simulink model "printer"  (R2017b)
settings: Solver=ode45  StartTime=0.0  StopTime=3  FixedStep=1e-4  MaxStep=1e-4  RelTol=1e-3  EnableMultiTasking=on
PreLoadFcn:
  | CONSTANTS
  | DEFAULT
  | System
  | Control
InitFcn:
  | CONSTANTS
  | DEFAULT
  | System
  | Control
values from neighbouring files (symbols this model uses):
  BackEMF0 = Q0(13)    [System.m]
  BackEMF1 = Q1(13)    [System.m]
  DegPerRad = 180/pi    (= 57.2957795131)    [CONSTANTS.m]    (also in kinematics_circle_MEGA.m = 57.3; kinematics_circle_fast_MEGA.m = 57.3; kinematics_circle_slow_MEGA.m = 57.3; kinematics_triangle_MEGA.m = 57.3)
  Elec0d = [Q0(11) Q0(10)]    [System.m]
  Elec0n = [1]    [System.m]
  Elec1d = [Q1(11) Q1(10)]    [System.m]
  Elec1n = [1]    [System.m]
  Height = 0.1    [CONSTANTS.m]
  Mech0d = [J0 B0]    [System.m]
  Mech0n = [1]    [System.m]
  Mech1d = [J1 B1]    [System.m]
  Mech1n = [1]    [System.m]
  NomI0 = Q0(6)    [System.m]
  NomI1 = Q1(6)    [System.m]
  PID0 = [0.178 8.83 0.0785]    [Control.m]
  PID1 = [Kp1 Ki1 Kd1]    [Control.m]
  StallI0 = Q0(8)    [System.m]
  StallI1 = Q1(8)    [System.m]
  StFric0 = 0.0024    [System.m]
  TConst0 = Q0(12)    [System.m]
  TConst1 = Q1(12)    [System.m]
undefined symbols (not defined in the file or in its folder): Amp1d, Amp1n, AmpSat1, JntSat1, Sens0, Sens1, SensSat0, SensSat1
libraries: simulink x14
settings Model: Creator=Leos  LastModifiedBy=cgx19
settings DataIOCC: SaveFormat=Array
settings OptimizationCC: ExpressionDepthLimit=2147483647  LifeSpan=inf
settings DebuggingCC: UnderspecifiedInitializationDetection=Classic  MergeDetectMultiDrivingBlocksExec=none  SolverPrmCheckMsg=warning  FcnCallInpInsideContextMsg=warning  StateNameClashWarn=warning  SFUnexpectedBacktrackingDiag=warning  SFNoUnconditionalDefaultTransitionDiag=warning  SFExecutionAtInitializationDiag=none
settings HardwareCC: ProdBitPerPointer=32  ProdBitPerSizeT=32  ProdBitPerPtrDiffT=32  ProdLargestAtomicFloat=None  ProdIntDivRoundTo=Undefined  ProdEndianess=Unspecified  ProdWordSize=32  ProdHWDeviceType=32-bit Generic
settings ModelReferenceCC: PropagateSignalLabelsOutOfModel=off
settings CodeAppCC: StateflowObjectComments=on
settings GRTTargetCC: TargetLangStandard=C89/C90 (ANSI)  GeneratePreprocessorConditionals=Disable all  CombineOutputUpdateFcns=off  GRTInterface=on
settings ConfigComp: CovMetricSettings=dw  CovHtmlReporting=on  CovSaveCumulativeToWorkspaceVar=on  CovSaveSingleToWorkspaceVar=on  CovExternalEMLEnable=off  CovSFcnEnable=off

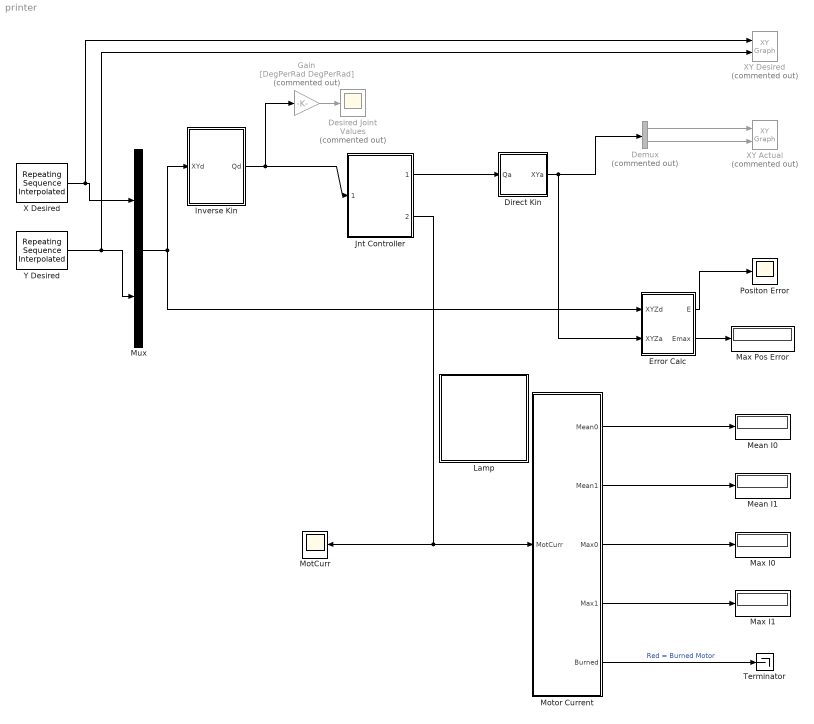
== system printer ==
  Demux : Demux  Commented=on  Outputs=2
  Desired Joint Values : Scope  Commented=on
  Direct Kin : Subsystem
  Error Calc : Subsystem
  Gain : Gain  Commented=on  Gain=[DegPerRad DegPerRad]
  Inverse Kin : Subsystem
  Jnt Controller : Subsystem
  Lamp : Subsystem  DialogController=hmiCreateDDGDialog  IsWebBlock=on  mask(MWDashboardBlock){webBlockId=7fcfd6b5-b98b-441a-9880-35fe4990fbef, webBlockType=lamp, ShowInLibBrowser=on, ShowInitialText=on, HMISrcModelName=printer}
      mask prompts: webBlockType "WebBlock Type"; HMISrcModelName "Source Model"
      mask help: SimulinkHMI:dialogs:LampDialogDesc
      mask Help: helpview([docroot '/mapfiles/simulink.map'], 'hmi_lamp')
      mask Display:
      | if strcmp(get_param(bdroot(gcb),'BlockDiagramType'), 'library')
      |     image([(matlabroot) '/toolbox/simulink/hmi/icons/Lamp.png']);
      | end
  Max I0 : Display
  Max I1 : Display
  Max Pos Error : Display
  Mean I0 : Display
  Mean I1 : Display
  MotCurr : Scope
  Motor Current : Subsystem
  Mux : Mux  Inputs=2
  Positon Error : Scope
  Terminator : Terminator
  X Desired : simulink/Sources/Repeating Sequence Interpolated  OutValues=Xd  TimeValues=Time  LookUpMeth=Interpolation-Use End Values  tsamp=SampleTime  OutMin=[]  OutMax=[]  OutDataTypeStr=double  OutputDataTypeScalingMode=double  OutDataType=fixdt(0,8)  OutScaling=2^-10
  XY Actual : simulink/Sinks/XY Graph  Commented=on  xmin=-125  xmax=125  ymin=-125  ymax=125  st=-1
  XY Desired : simulink/Sinks/XY Graph  Commented=on  xmin=-110  xmax=110  ymin=-110  ymax=110  st=-1
  Y Desired : simulink/Sources/Repeating Sequence Interpolated  OutValues=Yd  TimeValues=Time  LookUpMeth=Interpolation-Use End Values  tsamp=SampleTime  OutMin=[]  OutMax=[]  OutDataTypeStr=double  OutputDataTypeScalingMode=double  OutDataType=fixdt(0,8)  OutScaling=2^-10
  wires:
  Y Desired/1 -> XY Desired/2, Mux/2
  X Desired/1 -> Mux/1, XY Desired/1
  Demux/2 -> XY Actual/2
  Demux/1 -> XY Actual/1
  Inverse Kin/1(Qd) -> Jnt Controller/1(Qd(DiscAna)), Gain/1
  Mux/1 -> Error Calc/1(XYZd), Inverse Kin/1(XYd)
  Direct Kin/1(XYa) -> Error Calc/2(XYZa), Demux/1
  Error Calc/2(Emax) -> Max Pos Error/1
  Error Calc/1(E) -> Positon Error/1
  Jnt Controller/2(Motor Currents) -> MotCurr/1, Motor Current/1(MotCurr)
  Motor Current/1(Mean0) -> Mean I0/1
  Motor Current/4(Max1) -> Max I1/1
  Gain/1 -> Desired Joint Values/1
  Motor Current/3(Max0) -> Max I0/1
  Motor Current/2(Mean1) -> Mean I1/1
  Motor Current/5(Burned) -> Terminator/1  "Red = Burned Motor"
  Jnt Controller/1(Qa(ContAna)) -> Direct Kin/1(Qa)

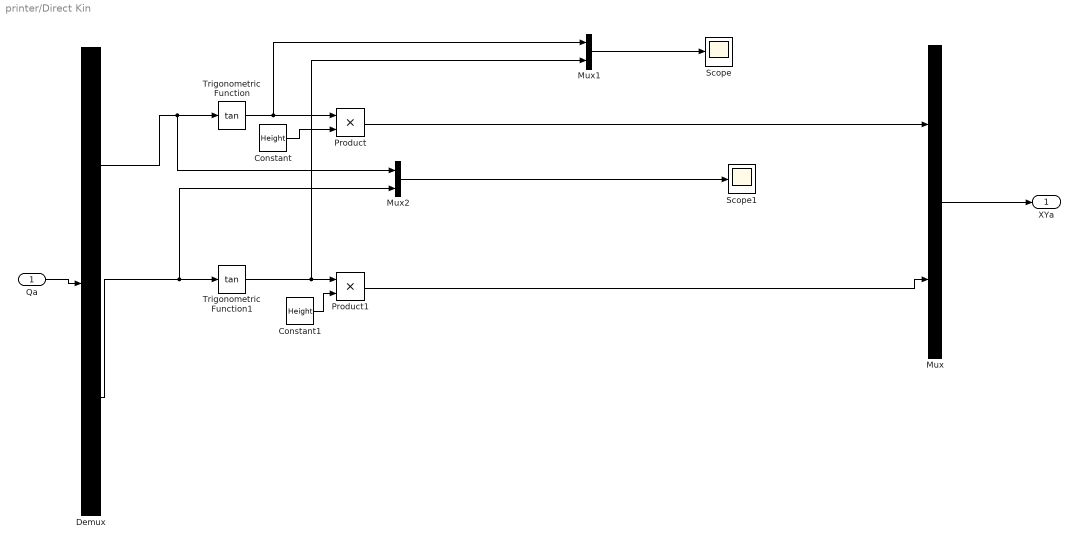
== system printer/Direct Kin ==
  Qa : Inport
  Constant : Constant  Value=Height
  Constant1 : Constant  Value=Height
  Demux : Demux  Outputs=2
  Mux : Mux  Inputs=2
  Mux1 : Mux  Inputs=2
  Mux2 : Mux  Inputs=2
  Product : Product
  Product1 : Product
  Scope : Scope
  Scope1 : Scope
  Trigonometric Function : Trigonometry  Operator=tan
  Trigonometric Function1 : Trigonometry  Operator=tan
  XYa : Outport
  wires:
  Qa/1 -> Demux/1
  Mux/1 -> XYa/1
  Demux/1 -> Mux2/1, Trigonometric Function/1
  Trigonometric Function/1 -> Mux1/1, Product/1
  Product/1 -> Mux/1
  Demux/2 -> Mux2/2, Trigonometric Function1/1
  Trigonometric Function1/1 -> Mux1/2, Product1/1
  Product1/1 -> Mux/2
  Mux1/1 -> Scope/1
  Mux2/1 -> Scope1/1
  Constant/1 -> Product/2
  Constant1/1 -> Product1/2

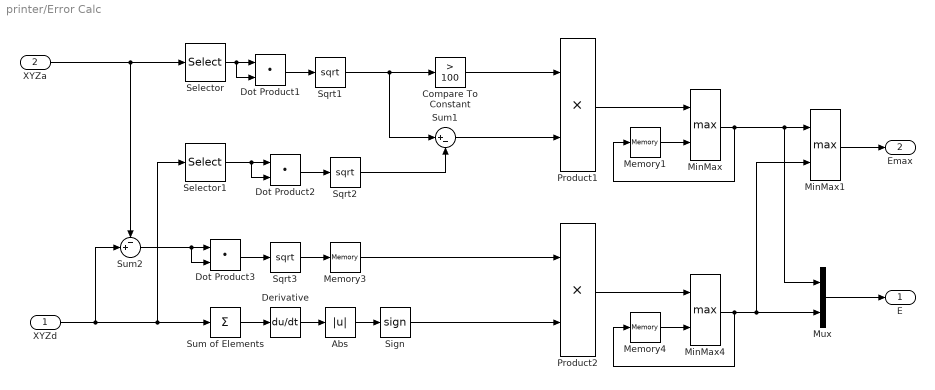
== system printer/Error Calc ==
  XYZd : Inport
  XYZa : Inport  Port=2
  Abs : Abs
  Compare To Constant : simulink/Logic and Bit Operations/Compare To Constant  relop=>  const=100  OutDataTypeStr=boolean
  Derivative : Derivative
  Dot Product1 : DotProduct  InputSameDT=on  OutDataTypeStr=Inherit: Inherit via internal rule
  Dot Product2 : DotProduct  InputSameDT=on  OutDataTypeStr=Inherit: Inherit via internal rule
  Dot Product3 : DotProduct  InputSameDT=on  OutDataTypeStr=Inherit: Inherit via internal rule
  Memory1 : Memory
  Memory3 : Memory
  Memory4 : Memory
  MinMax : MinMax  Function=max  Inputs=2
  MinMax1 : MinMax  Function=max  Inputs=2
  MinMax4 : MinMax  Function=max  Inputs=2
  Mux : Mux  Inputs=2
  Product1 : Product
  Product2 : Product
  Selector : Selector  InputPortWidth=2  IndexOptions=Index vector (dialog)  Indices=[1 2]  OutputSizes=1
  Selector1 : Selector  InputPortWidth=2  IndexOptions=Index vector (dialog)  Indices=[1 2]  OutputSizes=1
  Sign : Signum
  Sqrt1 : Sqrt  SaturateOnIntegerOverflow=on
  Sqrt2 : Sqrt  SaturateOnIntegerOverflow=on
  Sqrt3 : Sqrt  SaturateOnIntegerOverflow=on
  Sum of Elements : Sum  Inputs=+
  Sum1 : Sum  Inputs=|+-
  Sum2 : Sum  Inputs=-+|
  E : Outport
  Emax : Outport  Port=2
  wires:
  XYZd/1 -> Sum2/2, Selector1/1, Sum of Elements/1
  Derivative/1 -> Abs/1
  Abs/1 -> Sign/1
  Sum of Elements/1 -> Derivative/1
  Selector/1 -> Dot Product1/2, Dot Product1/1
  Dot Product1/1 -> Sqrt1/1
  XYZa/1 -> Sum2/1, Selector/1
  Sign/1 -> Product2/2
  Sqrt1/1 -> Sum1/1, Compare To Constant/1
  Product1/1 -> MinMax/1
  Compare To Constant/1 -> Product1/1
  Sum1/1 -> Product1/2
  Memory1/1 -> MinMax/2
  MinMax/1 -> Mux/1, MinMax1/1, Memory1/1
  Memory4/1 -> MinMax4/2
  Product2/1 -> MinMax4/1
  MinMax4/1 -> MinMax1/2, Mux/2, Memory4/1
  MinMax1/1 -> Emax/1
  Mux/1 -> E/1
  Memory3/1 -> Product2/1
  Selector1/1 -> Dot Product2/2, Dot Product2/1
  Dot Product2/1 -> Sqrt2/1
  Sqrt2/1 -> Sum1/2
  Sum2/1 -> Dot Product3/2, Dot Product3/1
  Dot Product3/1 -> Sqrt3/1
  Sqrt3/1 -> Memory3/1

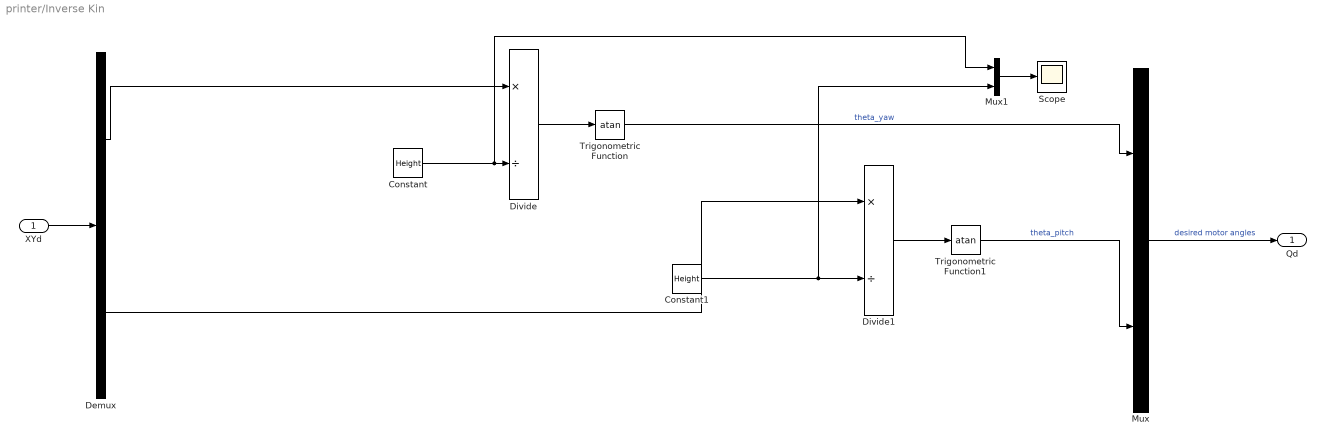
== system printer/Inverse Kin ==
  XYd : Inport
  Constant : Constant  Value=Height
  Constant1 : Constant  Value=Height
  Demux : Demux  Outputs=2
  Divide : Product  Inputs=*/
  Divide1 : Product  Inputs=*/
  Mux : Mux  Inputs=2
  Mux1 : Mux  Inputs=2
  Scope : Scope
  Trigonometric Function : Trigonometry  Operator=atan
  Trigonometric Function1 : Trigonometry  Operator=atan
  Qd : Outport
  wires:
  XYd/1 -> Demux/1
  Mux/1 -> Qd/1  "desired motor angles"
  Demux/2 -> Divide1/1
  Demux/1 -> Divide/1
  Divide/1 -> Trigonometric Function/1
  Divide1/1 -> Trigonometric Function1/1
  Constant1/1 -> Mux1/2, Divide1/2
  Constant/1 -> Mux1/1, Divide/2
  Trigonometric Function/1 -> Mux/1  "theta_yaw"
  Mux1/1 -> Scope/1
  Trigonometric Function1/1 -> Mux/2  "theta_pitch"

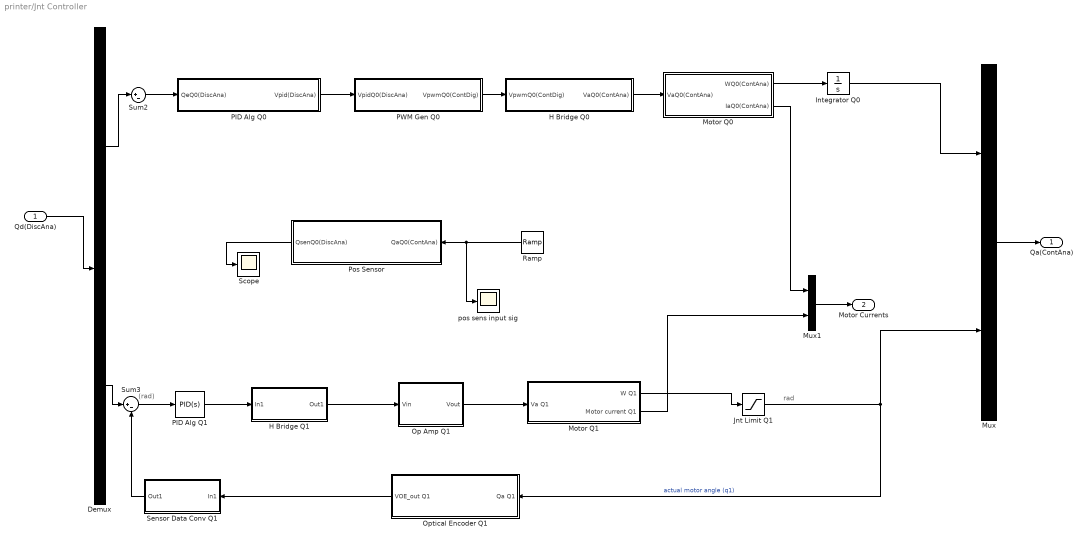
== system printer/Jnt Controller ==
  note: rad
  note: (rad)
  Qd(DiscAna) : Inport
  Demux : Demux  Outputs=2
  H Bridge Q0 : Subsystem
  H Bridge Q1 : Subsystem
  Integrator Q0 : Integrator
  Jnt Limit Q1 : Saturate  UpperLimit=JntSat1  LowerLimit=-JntSat1
  Motor Q0 : Subsystem
  Motor Q1 : Subsystem
  Mux : Mux  Inputs=2
  Mux1 : Mux  Inputs=2
  Op Amp Q1 : Subsystem
  Optical Encoder Q1 : Subsystem
  PID Alg Q1 : simulink/Continuous/PID Controller  Controller=PID  TimeDomain=Continuous-time  SampleTime=-1  IntegratorMethod=Forward Euler  FilterMethod=Forward Euler  Form=Parallel  UseFilter=on  ControllerParametersSource=internal  P=PID1(1)  I=PID1(2)  D=PID1(3)  N=100  InitialConditionSource=internal  InitialConditionForIntegrator=0  InitialConditionForFilter=0  ExternalReset=none  LimitOutput=off  UpperSaturationLimit=inf  LowerSaturationLimit=-inf  LinearizeAsGain=on  AntiWindupMode=none  Kb=1  TrackingMode=off  Kt=1  PParamMin=[]  PParamMax=[]  IParamMin=[]  IParamMax=[]  DParamMin=[]  DParamMax=[]  NParamMin=[]  NParamMax=[]  KbParamMin=[]  KbParamMax=[]  KtParamMin=[]  KtParamMax=[]  POutMin=[]  POutMax=[]  IOutMin=[]  IOutMax=[]  DOutMin=[]  DOutMax=[]  NOutMin=[]  NOutMax=[]  KbOutMin=[]  KbOutMax=[]  KtOutMin=[]  KtOutMax=[]  IntegratorOutMin=[]  IntegratorOutMax=[]  FilterOutMin=[]  FilterOutMax=[]  SumOutMin=[]  SumOutMax=[]  SumI1OutMin=[]  SumI1OutMax=[]  SumI2OutMin=[]  SumI2OutMax=[]  SumI3OutMin=[]  SumI3OutMax=[]  SumDOutMin=[]  SumDOutMax=[]  SaturationOutMin=[]  SaturationOutMax=[]  IntegratorContinuousStateAttributes=''  IntegratorStateMustResolveToSignalObject=off  IntegratorRTWStateStorageClass=Auto  FilterContinuousStateAttributes=''  FilterStateMustResolveToSignalObject=off  FilterRTWStateStorageClass=Auto  DifferentiatorICPrevScaledInput=0  DifferentiatorOutMin=[]  DifferentiatorOutMax=[]  InitialConditionSetting=State (most efficient)  FilterDiffOutCoefMin=[]  FilterDiffOutCoefMax=[]  SumDenOutMin=[]  SumDenOutMax=[]  SumNumOutMin=[]  SumNumOutMax=[]  ReciprocalOutMin=[]  ReciprocalOutMax=[]  DivideOutMin=[]  DivideOutMax=[]  TunerSelectOption=Transfer Function Based (PID Tuner App)
  PID Alg Q0 : Subsystem
  PWM Gen Q0 : Subsystem
  Pos Sensor : Subsystem
  Ramp : simulink/Sources/Ramp  slope=1  start=0  X0=0
  Scope : Scope
  Sensor Data Conv Q1 : Subsystem
  Sum2 : Sum  Inputs=|+-
  Sum3 : Sum  Inputs=|+-
  pos sens input sig : Scope
  Qa(ContAna) : Outport
  Motor Currents : Outport  Port=2
  wires:
  Qd(DiscAna)/1 -> Demux/1
  Mux/1 -> Qa(ContAna)/1
  Sum3/1 -> PID Alg Q1/1
  Demux/1 -> Sum2/1
  Demux/2 -> Sum3/1
  Sensor Data Conv Q1/1(Out1) -> Sum3/2
  Integrator Q0/1 -> Mux/1
  Jnt Limit Q1/1 -> Optical Encoder Q1/1(Qa Q1), Mux/2  "actual motor angle (q1)"
  Motor Q0/1(WQ0(ContAna)) -> Integrator Q0/1
  Motor Q1/1(W Q1) -> Jnt Limit Q1/1
  Motor Q0/2(IaQ0(ContAna)) -> Mux1/1
  Motor Q1/2(Motor current Q1) -> Mux1/2
  Mux1/1 -> Motor Currents/1
  Op Amp Q1/1(Vout) -> Motor Q1/1(Va Q1)
  PID Alg Q1/1 -> H Bridge Q1/1(In1)
  H Bridge Q1/1(Out1) -> Op Amp Q1/1(Vin)
  Optical Encoder Q1/1(VOE_out Q1) -> Sensor Data Conv Q1/1(In1)
  H Bridge Q0/1(VaQ0(ContAna)) -> Motor Q0/1(VaQ0(ContAna))
  PWM Gen Q0/1(VpwmQ0(ContDig)) -> H Bridge Q0/1("VpwmQ0(ContDig) ")
  Sum2/1 -> PID Alg Q0/1(QeQ0(DiscAna))
  PID Alg Q0/1(Vpid(DiscAna)) -> PWM Gen Q0/1(VpidQ0(DiscAna))
  Ramp/1 -> Pos Sensor/1(QaQ0(ContAna)), pos sens input sig/1
  Pos Sensor/1(QsenQ0(DiscAna)) -> Scope/1

== system printer/Lamp ==

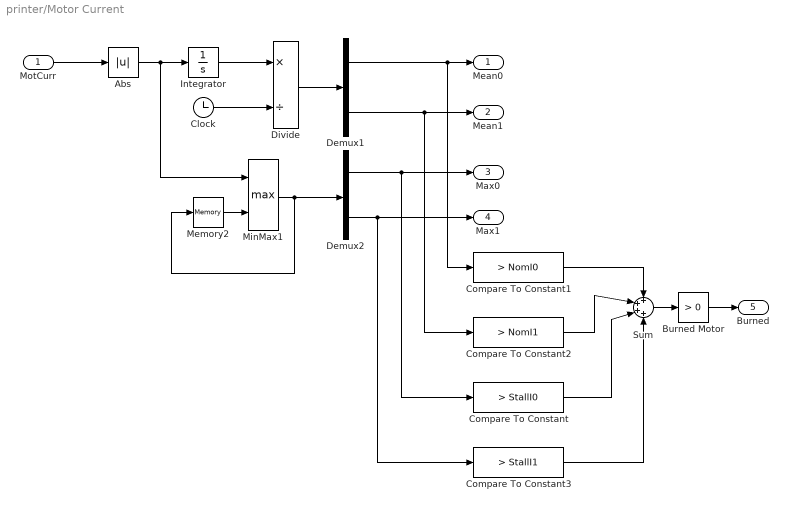
== system printer/Motor Current ==
  MotCurr : Inport
  Abs : Abs
  Burned Motor : simulink/Logic and Bit Operations/Compare To Zero  relop=>  OutDataTypeStr=boolean
  Clock : Clock
  Compare To Constant : simulink/Logic and Bit Operations/Compare To Constant  relop=>  const=StallI0  OutDataTypeStr=boolean
  Compare To Constant1 : simulink/Logic and Bit Operations/Compare To Constant  relop=>  const=NomI0  OutDataTypeStr=boolean
  Compare To Constant2 : simulink/Logic and Bit Operations/Compare To Constant  relop=>  const=NomI1  OutDataTypeStr=boolean
  Compare To Constant3 : simulink/Logic and Bit Operations/Compare To Constant  relop=>  const=StallI1  OutDataTypeStr=boolean
  Demux1 : Demux  Outputs=2
  Demux2 : Demux  Outputs=2
  Divide : Product  Inputs=*/
  Integrator : Integrator
  Memory2 : Memory
  MinMax1 : MinMax  Function=max  Inputs=2
  Sum : Sum  Inputs=++++
  Mean0 : Outport
  Mean1 : Outport  Port=2
  Max0 : Outport  Port=3
  Max1 : Outport  Port=4
  Burned : Outport  Port=5
  wires:
  Demux1/1 -> Compare To Constant1/1, Mean0/1
  MotCurr/1 -> Abs/1
  Integrator/1 -> Divide/1
  Clock/1 -> Divide/2
  Divide/1 -> Demux1/1
  Abs/1 -> MinMax1/1, Integrator/1
  Demux2/1 -> Compare To Constant/1, Max0/1
  Demux1/2 -> Compare To Constant2/1, Mean1/1
  Demux2/2 -> Compare To Constant3/1, Max1/1
  Compare To Constant1/1 -> Sum/1
  Compare To Constant3/1 -> Sum/4
  Compare To Constant/1 -> Sum/3
  Compare To Constant2/1 -> Sum/2
  Memory2/1 -> MinMax1/2
  MinMax1/1 -> Demux2/1, Memory2/1
  Burned Motor/1 -> Burned/1
  Sum/1 -> Burned Motor/1

== system printer/Jnt Controller/H Bridge Q0 ==
  "VpwmQ0(ContDig) " : Inport
  VaQ0(ContAna) : Outport
  wires:
  "VpwmQ0(ContDig) "/1 -> VaQ0(ContAna)/1

== system printer/Jnt Controller/H Bridge Q1 ==
  In1 : Inport
  Out1 : Outport
  wires:
  In1/1 -> Out1/1

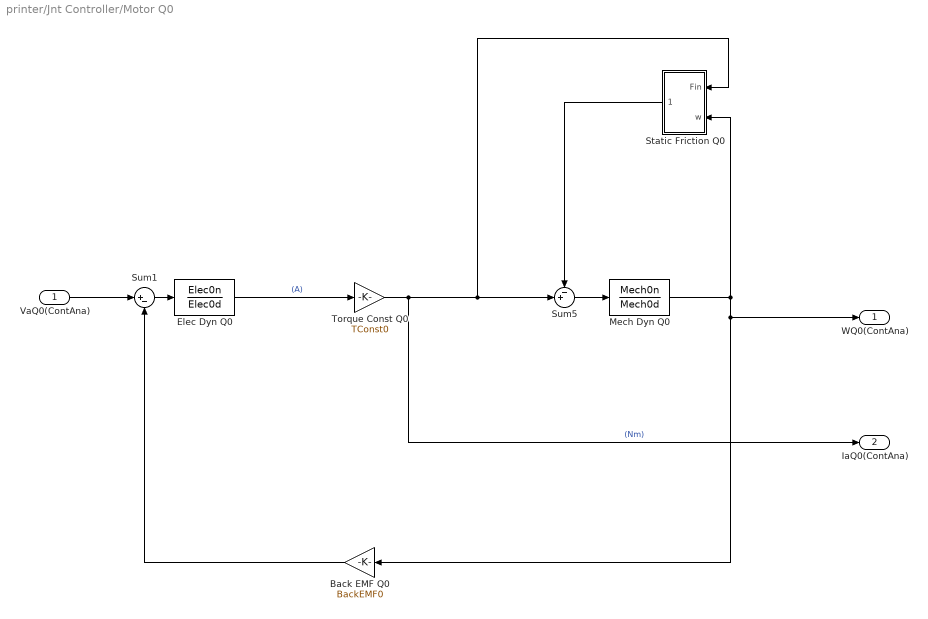
== system printer/Jnt Controller/Motor Q0 ==
  VaQ0(ContAna) : Inport
  Back EMF Q0 : Gain  Gain=BackEMF0
  Elec Dyn Q0 : TransferFcn  Numerator=Elec0n  Denominator=Elec0d
  Mech Dyn Q0 : TransferFcn  Numerator=Mech0n  Denominator=Mech0d
  Static Friction Q0 : Subsystem
  Sum1 : Sum  Inputs=|+-
  Sum5 : Sum  Inputs=-+|
  Torque Const Q0 : Gain  Gain=TConst0
  WQ0(ContAna) : Outport
  IaQ0(ContAna) : Outport  Port=2
  wires:
  Torque Const Q0/1 -> IaQ0(ContAna)/1, Sum5/2, Static Friction Q0/1(Fin)  "(Nm)"
  Sum5/1 -> Mech Dyn Q0/1
  Back EMF Q0/1 -> Sum1/2
  VaQ0(ContAna)/1 -> Sum1/1
  Elec Dyn Q0/1 -> Torque Const Q0/1  "(A)"
  Sum1/1 -> Elec Dyn Q0/1
  Mech Dyn Q0/1 -> Back EMF Q0/1, WQ0(ContAna)/1, Static Friction Q0/2(w)
  Static Friction Q0/1(Fout) -> Sum5/1

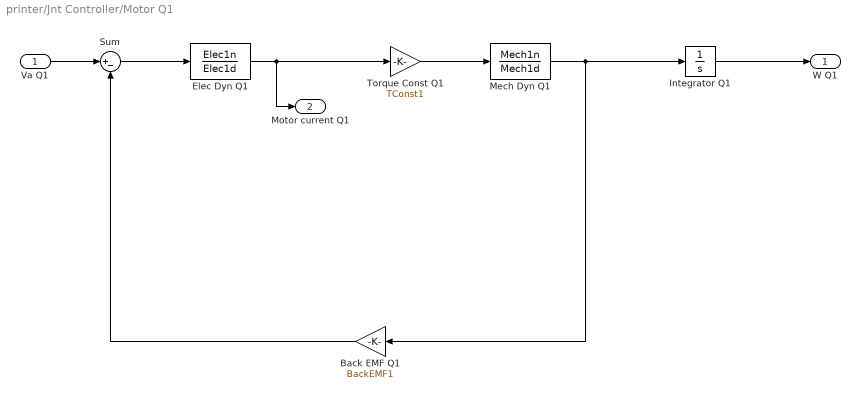
== system printer/Jnt Controller/Motor Q1 ==
  Va Q1 : Inport
  Back EMF Q1 : Gain  Gain=BackEMF1
  Elec Dyn Q1 : TransferFcn  Numerator=Elec1n  Denominator=Elec1d
  Integrator Q1 : Integrator
  Mech Dyn Q1 : TransferFcn  Numerator=Mech1n  Denominator=Mech1d
  Sum : Sum  Inputs=|+-
  Torque Const Q1 : Gain  Gain=TConst1
  W Q1 : Outport
  Motor current Q1 : Outport  Port=2
  wires:
  Sum/1 -> Elec Dyn Q1/1
  Back EMF Q1/1 -> Sum/2
  Elec Dyn Q1/1 -> Motor current Q1/1, Torque Const Q1/1
  Torque Const Q1/1 -> Mech Dyn Q1/1
  Integrator Q1/1 -> W Q1/1
  Mech Dyn Q1/1 -> Integrator Q1/1, Back EMF Q1/1
  Va Q1/1 -> Sum/1

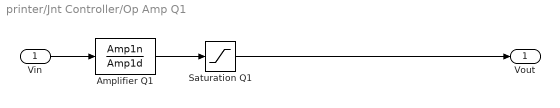
== system printer/Jnt Controller/Op Amp Q1 ==
  Vin : Inport
  Amplifier Q1 : TransferFcn  Numerator=Amp1n  Denominator=Amp1d
  Saturation Q1 : Saturate  UpperLimit=AmpSat1  LowerLimit=-AmpSat1
  Vout : Outport
  wires:
  Vin/1 -> Amplifier Q1/1
  Amplifier Q1/1 -> Saturation Q1/1
  Saturation Q1/1 -> Vout/1

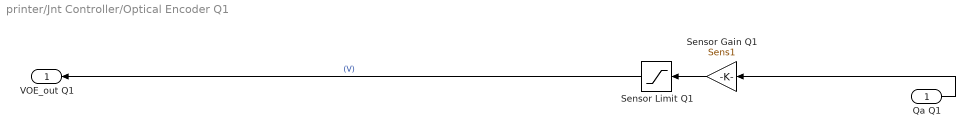
== system printer/Jnt Controller/Optical Encoder Q1 ==
  Qa Q1 : Inport
  Sensor Gain Q1 : Gain  Gain=Sens1
  Sensor Limit Q1 : Saturate  UpperLimit=SensSat1  LowerLimit=-SensSat1
  VOE_out Q1 : Outport
  wires:
  Sensor Gain Q1/1 -> Sensor Limit Q1/1
  Sensor Limit Q1/1 -> VOE_out Q1/1  "(V)"
  Qa Q1/1 -> Sensor Gain Q1/1

== system printer/Jnt Controller/PID Alg Q0 ==
  QeQ0(DiscAna) : Inport
  PID : simulink/Continuous/PID Controller  Controller=PID  TimeDomain=Continuous-time  SampleTime=-1  IntegratorMethod=Forward Euler  FilterMethod=Forward Euler  Form=Parallel  UseFilter=on  ControllerParametersSource=internal  P=PID0(1)  I=PID0(2)  D=PID0(3)  N=100  InitialConditionSource=internal  InitialConditionForIntegrator=0  InitialConditionForFilter=0  ExternalReset=none  LimitOutput=off  UpperSaturationLimit=inf  LowerSaturationLimit=-inf  LinearizeAsGain=on  AntiWindupMode=none  Kb=1  TrackingMode=off  Kt=1  PParamMin=[]  PParamMax=[]  IParamMin=[]  IParamMax=[]  DParamMin=[]  DParamMax=[]  NParamMin=[]  NParamMax=[]  KbParamMin=[]  KbParamMax=[]  KtParamMin=[]  KtParamMax=[]  POutMin=[]  POutMax=[]  IOutMin=[]  IOutMax=[]  DOutMin=[]  DOutMax=[]  NOutMin=[]  NOutMax=[]  KbOutMin=[]  KbOutMax=[]  KtOutMin=[]  KtOutMax=[]  IntegratorOutMin=[]  IntegratorOutMax=[]  FilterOutMin=[]  FilterOutMax=[]  SumOutMin=[]  SumOutMax=[]  SumI1OutMin=[]  SumI1OutMax=[]  SumI2OutMin=[]  SumI2OutMax=[]  SumI3OutMin=[]  SumI3OutMax=[]  SumDOutMin=[]  SumDOutMax=[]  SaturationOutMin=[]  SaturationOutMax=[]  IntegratorContinuousStateAttributes=''  IntegratorStateMustResolveToSignalObject=off  IntegratorRTWStateStorageClass=Auto  FilterContinuousStateAttributes=''  FilterStateMustResolveToSignalObject=off  FilterRTWStateStorageClass=Auto  DifferentiatorICPrevScaledInput=0  DifferentiatorOutMin=[]  DifferentiatorOutMax=[]  InitialConditionSetting=State (most efficient)  FilterDiffOutCoefMin=[]  FilterDiffOutCoefMax=[]  SumDenOutMin=[]  SumDenOutMax=[]  SumNumOutMin=[]  SumNumOutMax=[]  ReciprocalOutMin=[]  ReciprocalOutMax=[]  DivideOutMin=[]  DivideOutMax=[]  TunerSelectOption=Transfer Function Based (PID Tuner App)
  Vpid(DiscAna) : Outport
  wires:
  QeQ0(DiscAna)/1 -> PID/1
  PID/1 -> Vpid(DiscAna)/1

== system printer/Jnt Controller/PWM Gen Q0 ==
  VpidQ0(DiscAna) : Inport
  VpwmQ0(ContDig) : Outport
  wires:
  VpidQ0(DiscAna)/1 -> VpwmQ0(ContDig)/1

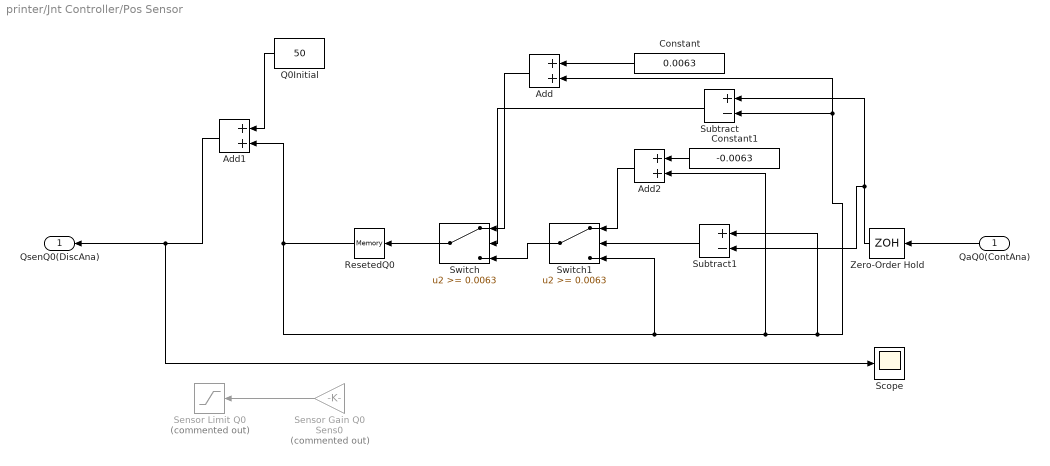
== system printer/Jnt Controller/Pos Sensor ==
  QaQ0(ContAna) : Inport
  Add : Sum
  Add1 : Sum
  Add2 : Sum
  Constant : Constant  Value=0.0063
  Constant1 : Constant  Value=-0.0063
  Q0Initial : Constant  Value=50
  ResetedQ0 : Memory
  Scope : Scope
  Sensor Gain Q0 : Gain  Commented=on  Gain=Sens0
  Sensor Limit Q0 : Saturate  Commented=on  UpperLimit=SensSat0  LowerLimit=-SensSat0
  Subtract : Sum  Inputs=+-
  Subtract1 : Sum  Inputs=+-
  Switch : Switch  Threshold=0.0063
  Switch1 : Switch  Threshold=0.0063
  Zero-Order Hold : ZeroOrderHold  SampleTime=0.001
  QsenQ0(DiscAna) : Outport
  wires:
  QaQ0(ContAna)/1 -> Zero-Order Hold/1
  Sensor Gain Q0/1 -> Sensor Limit Q0/1
  Add1/1 -> Scope/1, QsenQ0(DiscAna)/1
  Q0Initial/1 -> Add1/1
  ResetedQ0/1 -> Switch1/3, Add2/2, Subtract1/1, Add/2, Subtract/2, Add1/2
  Zero-Order Hold/1 -> Subtract1/2, Subtract/1
  Subtract/1 -> Switch/2
  Constant/1 -> Add/1
  Add/1 -> Switch/1
  Constant1/1 -> Add2/1
  Switch1/1 -> Switch/3
  Add2/1 -> Switch1/1
  Subtract1/1 -> Switch1/2
  Switch/1 -> ResetedQ0/1

== system printer/Jnt Controller/Sensor Data Conv Q1 ==
  In1 : Inport
  Out1 : Outport
  wires:
  In1/1 -> Out1/1

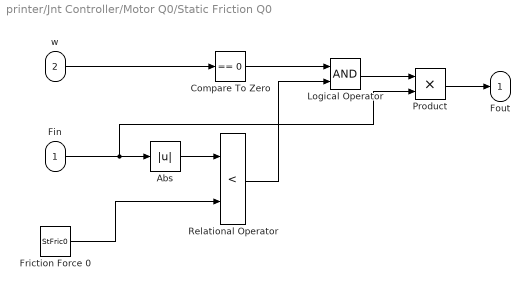
== system printer/Jnt Controller/Motor Q0/Static Friction Q0 ==
  Fin : Inport
  w : Inport  Port=2
  Abs : Abs
  Compare To Zero : simulink/Logic and Bit Operations/Compare To Zero  relop===  OutDataTypeStr=boolean
  Friction Force 0 : Constant  Value=StFric0
  Logical Operator : Logic  AllPortsSameDT=off  OutDataTypeStr=boolean
  Product : Product
  Relational Operator : RelationalOperator  Operator=<  OutDataTypeStr=boolean  RndMeth=Simplest
  Fout : Outport
  wires:
  Friction Force 0/1 -> Relational Operator/2
  Product/1 -> Fout/1
  Compare To Zero/1 -> Logical Operator/1
  Relational Operator/1 -> Logical Operator/2
  Logical Operator/1 -> Product/1
  Fin/1 -> Product/2, Abs/1
  w/1 -> Compare To Zero/1
  Abs/1 -> Relational Operator/1
